simulink model "Boost_Converter"  (R2023b)
settings: Solver=VariableStepAuto  StartTime=0.0  StopTime=2  RelTol=1e-3
libraries: spsSeriesRLCBranchLib x4, spsCurrentMeasurementLib x1, spsDCVoltageSourceLib x1, spsDiodeLib x1, spsIGBTDiodeLib x1, spsVoltageMeasurementLib x1, sps_lib x1
settings Model: Creator=Anusha  LastModifiedBy=Anusha

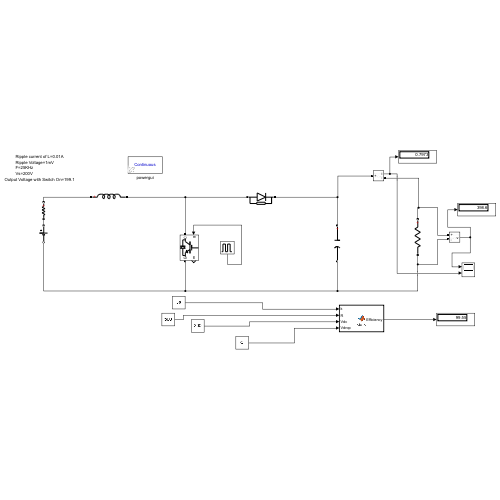
[thumbnail: Simulink's stored preview of the top-level diagram]
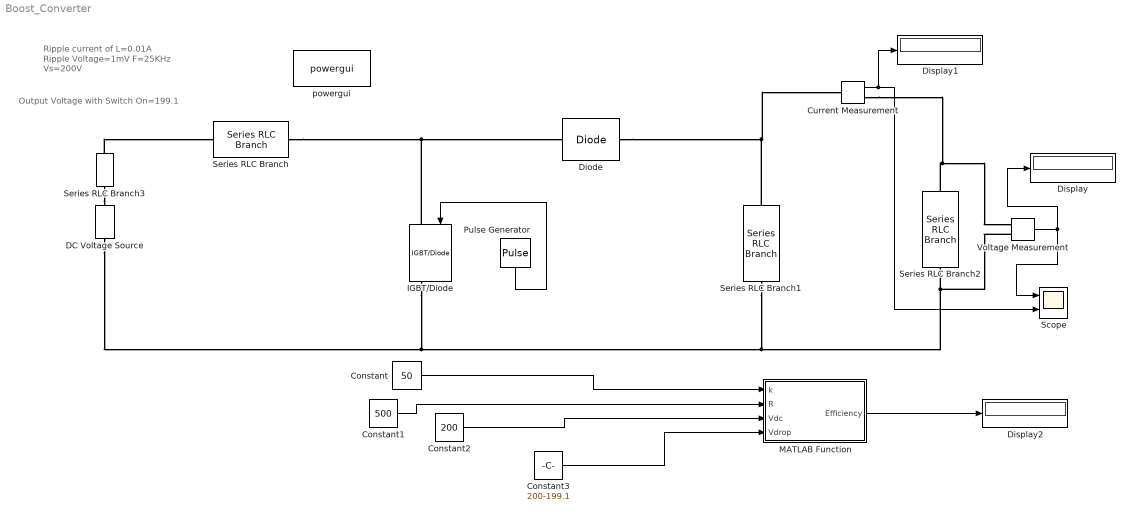
== system Boost_Converter ==
  note: Ripple current of L=0.01A
      | Ripple Voltage=1mV
      | F=25KHz
      | Vs=200V
  note: Output Voltage with Switch On=199.1
  Constant : Constant  Value=50
  Constant1 : Constant  Value=500
  Constant2 : Constant  Value=200
  Constant3 : Constant  Value=200-199.1
  Current Measurement : spsCurrentMeasurementLib/Current Measurement  PhasorSimulation=off  OutputType=Complex  PSBequivalent=0
  DC Voltage Source : spsDCVoltageSourceLib/DC Voltage Source  Amplitude=200  Measurements=None
  Diode : spsDiodeLib/Diode  Ron=0.001  Lon=0  Vf=0.8  IC=0  UseSnubber=0  Rs=500  Cs=250e-9  Measurements=off
  Display : Display
  Display1 : Display
  Display2 : Display
  IGBT/Diode : spsIGBTDiodeLib/IGBT//Diode  Ron=1e-3  Rs=1e5  Cs=inf  Measurements=on
  MATLAB Function : MATLAB Function  TreatAsAtomicUnit=on
  Pulse Generator : DiscretePulseGenerator  PulseType=Time based  Period=1/25000  PulseWidth=50
  Scope : Scope  NumInputPorts=2
  Series RLC Branch : spsSeriesRLCBranchLib/Series RLC Branch  LConnTagsString=__new0  RConnTagsString=__new0  BranchType=L  Resistance=1  Inductance=0.16  SetiL0=off  InitialCurrent=0  Capacitance=1e-6  Setx0=off  InitialVoltage=0  Measurements=None
  Series RLC Branch1 : spsSeriesRLCBranchLib/Series RLC Branch  LConnTagsString=__new0  RConnTagsString=__new0  BranchType=C  Resistance=1  Inductance=1e-3  SetiL0=off  InitialCurrent=0  Capacitance=50e-6  Setx0=off  InitialVoltage=0  Measurements=None
  Series RLC Branch2 : spsSeriesRLCBranchLib/Series RLC Branch  LConnTagsString=__new0  RConnTagsString=__new0  BranchType=R  Resistance=500  Inductance=1e-3  SetiL0=off  InitialCurrent=0  Capacitance=1e-6  Setx0=off  InitialVoltage=0  Measurements=None
  Series RLC Branch3 : spsSeriesRLCBranchLib/Series RLC Branch  LConnTagsString=__new0  RConnTagsString=__new0  BranchType=R  Resistance=0.2  Inductance=1e-3  SetiL0=off  InitialCurrent=0  Capacitance=1e-6  Setx0=off  InitialVoltage=0  Measurements=None
  Voltage Measurement : spsVoltageMeasurementLib/Voltage Measurement  PhasorSimulation=off  OutputType=Complex  PSBequivalent=0
  powergui : sps_lib/powergui  Priority=1  SimulationMode=Continuous  SampleTime=50e-6  frequency=60  Iterations=50  frequencyindice=0  Pbase=100e6  ErrMax=1e-4  UnitsV=kV  UnitsW=MW  buscounter=0  FunctionMessages=off  echomessages=off  EnableUseOfTLC=off  CurrentSourceSwitches=off  DisableSnubberDevices=off  DisableRonSwitches=off  DisableVfSwitches=off  DisplayEquations=off  AutomaticDiscreteSolvers=off  SolverType=Tustin/Backward Euler (TBE)  Interpol=off  ExternalGateDelay=off  methode=off  Ts=100  x0status=blocks  SPID=on  SwTol=0  HookPort=off  NonlinearTolerance=1e-4  nMaxIteration=100  ContinueOnMaxIteration=off  RestoreLinks=warning  ResistiveCurrentMeasurement=off  Frange=[0:2:500]  Ylog=off  Xlog=on  ShowGrid=off  save=off  variable=ZData  structure=0  ZoomFFT=off  StartTime=0.0  cycles=1  DisplayStyle=1  fundamental=60  FreqAxis=off  MaxFrequency=1000  frequencyindicesteady=1  RmsSteady=1  display=off
  wires:
  Pulse Generator/1 -> IGBT/Diode/1
  Constant2/1 -> MATLAB Function/3(Vdc)
  MATLAB Function/1(Efficiency) -> Display2/1
  Constant/1 -> MATLAB Function/1(k)
  Current Measurement/1 -> Display1/1, Scope/2
  Constant1/1 -> MATLAB Function/2(R)
  Constant3/1 -> MATLAB Function/4(Vdrop)
  Voltage Measurement/1 -> Display/1, Scope/1
  connections:
  Series RLC Branch2/RConn1 -- DC Voltage Source/LConn1 -- IGBT/Diode/RConn1 -- Series RLC Branch1/RConn1 -- Voltage Measurement/LConn2
  Series RLC Branch1/LConn1 -- Current Measurement/LConn1 -- Diode/RConn1
  Series RLC Branch2/LConn1 -- Current Measurement/RConn1 -- Voltage Measurement/LConn1
  Series RLC Branch3/RConn1 -- DC Voltage Source/RConn1
  Series RLC Branch3/LConn1 -- Series RLC Branch/LConn1
  Series RLC Branch/RConn1 -- IGBT/Diode/LConn1 -- Diode/LConn1

== matlab function Boost_Converter/MATLAB Function ==
  data: k input; Efficiency output; R input; Vdc input; Vdrop input
function Efficiency = stats(k,R,Vdc,Vdrop)

Po=k*((Vdc-Vdrop).^2)/R;
Pi=k*((Vdc-Vdrop)*Vdc)/R;
Efficiency=(Po/Pi)*100
